simulink model "REL_TestModel"  (R2022a)
settings: Solver=FixedStepDiscrete  StartTime=0.0  StopTime=10.0  FixedStep=0.01  RelTol=1e-3
settings Model: DataDictionary=DHM.sldd  Creator=DELL  LastModifiedBy=DELL
settings DataIOCC: SaveFormat=StructureWithTime
settings OptimizationCC: DefaultParameterBehavior=Inlined  EnhancedBackFolding=on  PassReuseOutputArgsAs=Individual arguments  ZeroExternalMemoryAtStartup=off  ZeroInternalMemoryAtStartup=off  OptimizeBlockOrder=speed  DifferentSizesBufferReuse=on  OptimizationCustomize=off  EfficientTunableParamExpr=on
settings DebuggingCC: ParameterTunabilityLossMsg=error
settings ModelReferenceCC: ModelReferenceNumInstancesAllowed=Single
settings SFSimCC: MATLABDynamicMemAlloc=off
settings RTWCC: Description=AUTOSAR  SystemTargetFile=autosar.tlc  GenCodeOnly=on  TemplateMakefile=ert_default_tmf
settings CodeAppCC: ForceParamTrailComments=on  IgnoreCustomStorageClasses=off  OperatorAnnotations=on  SimulinkDataObjDesc=on  SFDataObjDesc=on  InsertBlockDesc=on
settings STFCustomTargetCC: TargetLangStandard=C99 (ISO)  MultiwordLength=256  ParMdlRefBuildCompliant=on  CompOptLevelCompliant=on  IncludeMdlTerminateFcn=off  CombineOutputUpdateFcns=on  SuppressErrorStatus=on  ERTCustomFileBanners=on  SupportNonFinite=off  SupportComplex=off  SupportContinuousTime=off  SupportNonInlinedSFcns=off  RemoveResetFunc=on  MATLABClassNameForMDSCustomization=Simulink.SoftwareTarget.ERTCustomization  AutosarCompliant=on  GRTInterface=off  UseToolchainInfoCompliant=on  LookupTableObjectStructAxisOrder=2,1,3,4,...  LUTObjectStructOrderEvenSpacing=Size,Table,Breakpoints  SystemTargetFile=autosar.tlc
settings ERTTargetCC: TargetLangStandard=C99 (ISO)  ConcurrentExecutionCompliant=off  IncludeMdlTerminateFcn=off  SuppressErrorStatus=on  SupportNonFinite=off  SupportComplex=off  ModelStepFunctionPrototypeControlCompliant=off  CPPClassGenCompliant=off  AutosarCompliant=on  LookupTableObjectStructAxisOrder=2,1,3,4,...  LUTObjectStructOrderEvenSpacing=Size,Table,Breakpoints  InlinedParameterPlacement=NonHierarchical  ERTCustomFileTemplate=example_file_process.tlc

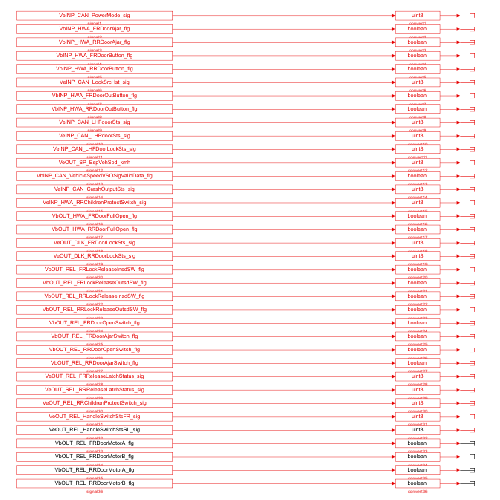
[thumbnail: Simulink's stored preview of the top-level diagram]
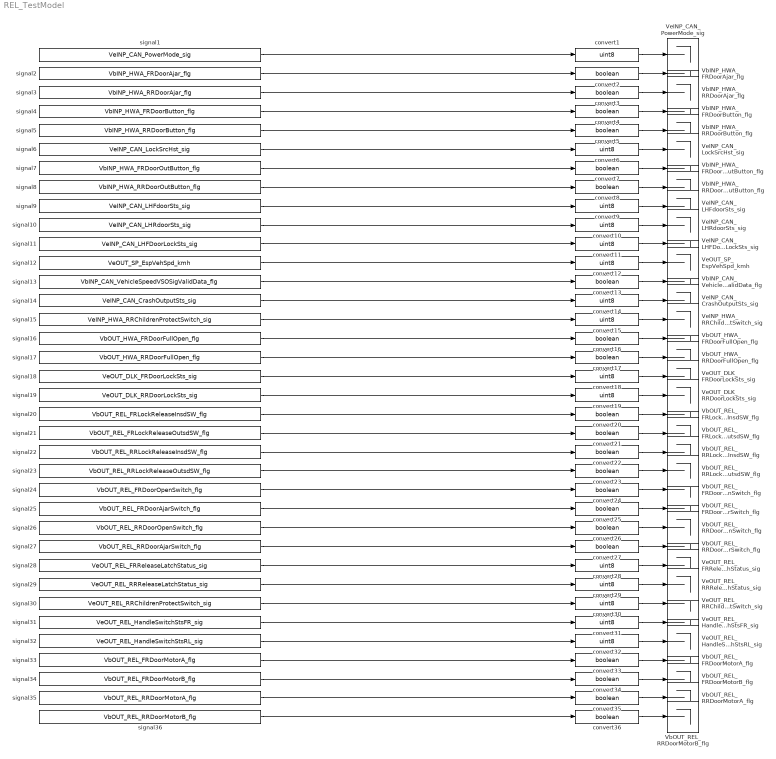
== system REL_TestModel ==
  VbINP_CAN_VehicleSpeedVSOSigValidData_flg : Terminator
  VbINP_HWA_FRDoorAjar_flg : Terminator
  VbINP_HWA_FRDoorButton_flg : Terminator
  VbINP_HWA_FRDoorOutButton_flg : Terminator
  VbINP_HWA_RRDoorAjar_flg : Terminator
  VbINP_HWA_RRDoorButton_flg : Terminator
  VbINP_HWA_RRDoorOutButton_flg : Terminator
  VbOUT_HWA_FRDoorFullOpen_flg : Terminator
  VbOUT_HWA_RRDoorFullOpen_flg : Terminator
  VbOUT_REL_FRDoorAjarSwitch_flg : Terminator
  VbOUT_REL_FRDoorMotorA_flg : Terminator
  VbOUT_REL_FRDoorMotorB_flg : Terminator
  VbOUT_REL_FRDoorOpenSwitch_flg : Terminator
  VbOUT_REL_FRLockReleaseInsdSW_flg : Terminator
  VbOUT_REL_FRLockReleaseOutsdSW_flg : Terminator
  VbOUT_REL_RRDoorAjarSwitch_flg : Terminator
  VbOUT_REL_RRDoorMotorA_flg : Terminator
  VbOUT_REL_RRDoorMotorB_flg : Terminator
  VbOUT_REL_RRDoorOpenSwitch_flg : Terminator
  VbOUT_REL_RRLockReleaseInsdSW_flg : Terminator
  VbOUT_REL_RRLockReleaseOutsdSW_flg : Terminator
  VeINP_CAN_CrashOutputSts_sig : Terminator
  VeINP_CAN_LHFDoorLockSts_sig : Terminator
  VeINP_CAN_LHFdoorSts_sig : Terminator
  VeINP_CAN_LHRdoorSts_sig : Terminator
  VeINP_CAN_LockSrcHst_sig : Terminator
  VeINP_CAN_PowerMode_sig : Terminator
  VeINP_HWA_RRChildrenProtectSwitch_sig : Terminator
  VeOUT_DLK_FRDoorLockSts_sig : Terminator
  VeOUT_DLK_RRDoorLockSts_sig : Terminator
  VeOUT_REL_FRReleaseLatchStatus_sig : Terminator
  VeOUT_REL_HandleSwitchStsFR_sig : Terminator
  VeOUT_REL_HandleSwitchStsRL_sig : Terminator
  VeOUT_REL_RRChildrenProtectSwitch_sig : Terminator
  VeOUT_REL_RRReleaseLatchStatus_sig : Terminator
  VeOUT_SP_EspVehSpd_kmh : Terminator
  convert{1,6,9..12,14..15,18..19,28..32} (15 alike) : DataTypeConversion  OutDataTypeStr=uint8  SaturateOnIntegerOverflow=off  RndMeth=Floor
  convert{2..5,7..8,13,16..17,20..27,33..36} (21 alike) : DataTypeConversion  OutDataTypeStr=boolean  SaturateOnIntegerOverflow=off  RndMeth=Floor
  signal1 : FromWorkspace  VariableName=VeINP_CAN_PowerMode_sig  SampleTime=-1  Interpolate=off  OutputAfterFinalValue=Holding final value
  signal10 : FromWorkspace  VariableName=VeINP_CAN_LHRdoorSts_sig  SampleTime=-1  Interpolate=off  OutputAfterFinalValue=Holding final value
  signal11 : FromWorkspace  VariableName=VeINP_CAN_LHFDoorLockSts_sig  SampleTime=-1  Interpolate=off  OutputAfterFinalValue=Holding final value
  signal12 : FromWorkspace  VariableName=VeOUT_SP_EspVehSpd_kmh  SampleTime=-1  Interpolate=off  OutputAfterFinalValue=Holding final value
  signal13 : FromWorkspace  VariableName=VbINP_CAN_VehicleSpeedVSOSigValidData_flg  SampleTime=-1  Interpolate=off  OutputAfterFinalValue=Holding final value
  signal14 : FromWorkspace  VariableName=VeINP_CAN_CrashOutputSts_sig  SampleTime=-1  Interpolate=off  OutputAfterFinalValue=Holding final value
  signal15 : FromWorkspace  VariableName=VeINP_HWA_RRChildrenProtectSwitch_sig  SampleTime=-1  Interpolate=off  OutputAfterFinalValue=Holding final value
  signal16 : FromWorkspace  VariableName=VbOUT_HWA_FRDoorFullOpen_flg  SampleTime=-1  Interpolate=off  OutputAfterFinalValue=Holding final value
  signal17 : FromWorkspace  VariableName=VbOUT_HWA_RRDoorFullOpen_flg  SampleTime=-1  Interpolate=off  OutputAfterFinalValue=Holding final value
  signal18 : FromWorkspace  VariableName=VeOUT_DLK_FRDoorLockSts_sig  SampleTime=-1  Interpolate=off  OutputAfterFinalValue=Holding final value
  signal19 : FromWorkspace  VariableName=VeOUT_DLK_RRDoorLockSts_sig  SampleTime=-1  Interpolate=off  OutputAfterFinalValue=Holding final value
  signal2 : FromWorkspace  VariableName=VbINP_HWA_FRDoorAjar_flg  SampleTime=-1  Interpolate=off  OutputAfterFinalValue=Holding final value
  signal20 : FromWorkspace  VariableName=VbOUT_REL_FRLockReleaseInsdSW_flg  SampleTime=-1  Interpolate=off  OutputAfterFinalValue=Holding final value
  signal21 : FromWorkspace  VariableName=VbOUT_REL_FRLockReleaseOutsdSW_flg  SampleTime=-1  Interpolate=off  OutputAfterFinalValue=Holding final value
  signal22 : FromWorkspace  VariableName=VbOUT_REL_RRLockReleaseInsdSW_flg  SampleTime=-1  Interpolate=off  OutputAfterFinalValue=Holding final value
  signal23 : FromWorkspace  VariableName=VbOUT_REL_RRLockReleaseOutsdSW_flg  SampleTime=-1  Interpolate=off  OutputAfterFinalValue=Holding final value
  signal24 : FromWorkspace  VariableName=VbOUT_REL_FRDoorOpenSwitch_flg  SampleTime=-1  Interpolate=off  OutputAfterFinalValue=Holding final value
  signal25 : FromWorkspace  VariableName=VbOUT_REL_FRDoorAjarSwitch_flg  SampleTime=-1  Interpolate=off  OutputAfterFinalValue=Holding final value
  signal26 : FromWorkspace  VariableName=VbOUT_REL_RRDoorOpenSwitch_flg  SampleTime=-1  Interpolate=off  OutputAfterFinalValue=Holding final value
  signal27 : FromWorkspace  VariableName=VbOUT_REL_RRDoorAjarSwitch_flg  SampleTime=-1  Interpolate=off  OutputAfterFinalValue=Holding final value
  signal28 : FromWorkspace  VariableName=VeOUT_REL_FRReleaseLatchStatus_sig  SampleTime=-1  Interpolate=off  OutputAfterFinalValue=Holding final value
  signal29 : FromWorkspace  VariableName=VeOUT_REL_RRReleaseLatchStatus_sig  SampleTime=-1  Interpolate=off  OutputAfterFinalValue=Holding final value
  signal3 : FromWorkspace  VariableName=VbINP_HWA_RRDoorAjar_flg  SampleTime=-1  Interpolate=off  OutputAfterFinalValue=Holding final value
  signal30 : FromWorkspace  VariableName=VeOUT_REL_RRChildrenProtectSwitch_sig  SampleTime=-1  Interpolate=off  OutputAfterFinalValue=Holding final value
  signal31 : FromWorkspace  VariableName=VeOUT_REL_HandleSwitchStsFR_sig  SampleTime=-1  Interpolate=off  OutputAfterFinalValue=Holding final value
  signal32 : FromWorkspace  VariableName=VeOUT_REL_HandleSwitchStsRL_sig  SampleTime=-1  Interpolate=off  OutputAfterFinalValue=Holding final value
  signal33 : FromWorkspace  VariableName=VbOUT_REL_FRDoorMotorA_flg  SampleTime=-1  Interpolate=off  OutputAfterFinalValue=Holding final value
  signal34 : FromWorkspace  VariableName=VbOUT_REL_FRDoorMotorB_flg  SampleTime=-1  Interpolate=off  OutputAfterFinalValue=Holding final value
  signal35 : FromWorkspace  VariableName=VbOUT_REL_RRDoorMotorA_flg  SampleTime=-1  Interpolate=off  OutputAfterFinalValue=Holding final value
  signal36 : FromWorkspace  VariableName=VbOUT_REL_RRDoorMotorB_flg  SampleTime=-1  Interpolate=off  OutputAfterFinalValue=Holding final value
  signal4 : FromWorkspace  VariableName=VbINP_HWA_FRDoorButton_flg  SampleTime=-1  Interpolate=off  OutputAfterFinalValue=Holding final value
  signal5 : FromWorkspace  VariableName=VbINP_HWA_RRDoorButton_flg  SampleTime=-1  Interpolate=off  OutputAfterFinalValue=Holding final value
  signal6 : FromWorkspace  VariableName=VeINP_CAN_LockSrcHst_sig  SampleTime=-1  Interpolate=off  OutputAfterFinalValue=Holding final value
  signal7 : FromWorkspace  VariableName=VbINP_HWA_FRDoorOutButton_flg  SampleTime=-1  Interpolate=off  OutputAfterFinalValue=Holding final value
  signal8 : FromWorkspace  VariableName=VbINP_HWA_RRDoorOutButton_flg  SampleTime=-1  Interpolate=off  OutputAfterFinalValue=Holding final value
  signal9 : FromWorkspace  VariableName=VeINP_CAN_LHFdoorSts_sig  SampleTime=-1  Interpolate=off  OutputAfterFinalValue=Holding final value
  wires:
  signal1/1 -> convert1/1
  signal2/1 -> convert2/1
  signal3/1 -> convert3/1
  signal4/1 -> convert4/1
  signal5/1 -> convert5/1
  signal6/1 -> convert6/1
  signal7/1 -> convert7/1
  signal8/1 -> convert8/1
  signal9/1 -> convert9/1
  signal10/1 -> convert10/1
  signal11/1 -> convert11/1
  signal12/1 -> convert12/1
  signal13/1 -> convert13/1
  signal14/1 -> convert14/1
  signal15/1 -> convert15/1
  signal16/1 -> convert16/1
  signal17/1 -> convert17/1
  signal18/1 -> convert18/1
  signal19/1 -> convert19/1
  signal20/1 -> convert20/1
  signal21/1 -> convert21/1
  signal22/1 -> convert22/1
  signal23/1 -> convert23/1
  signal24/1 -> convert24/1
  signal25/1 -> convert25/1
  signal26/1 -> convert26/1
  signal27/1 -> convert27/1
  signal28/1 -> convert28/1
  signal29/1 -> convert29/1
  signal30/1 -> convert30/1
  signal31/1 -> convert31/1
  signal32/1 -> convert32/1
  signal33/1 -> convert33/1
  signal34/1 -> convert34/1
  signal35/1 -> convert35/1
  signal36/1 -> convert36/1
  convert1/1 -> VeINP_CAN_PowerMode_sig/1
  convert10/1 -> VeINP_CAN_LHRdoorSts_sig/1
  convert11/1 -> VeINP_CAN_LHFDoorLockSts_sig/1
  convert12/1 -> VeOUT_SP_EspVehSpd_kmh/1
  convert13/1 -> VbINP_CAN_VehicleSpeedVSOSigValidData_flg/1
  convert14/1 -> VeINP_CAN_CrashOutputSts_sig/1
  convert15/1 -> VeINP_HWA_RRChildrenProtectSwitch_sig/1
  convert16/1 -> VbOUT_HWA_FRDoorFullOpen_flg/1
  convert17/1 -> VbOUT_HWA_RRDoorFullOpen_flg/1
  convert18/1 -> VeOUT_DLK_FRDoorLockSts_sig/1
  convert19/1 -> VeOUT_DLK_RRDoorLockSts_sig/1
  convert2/1 -> VbINP_HWA_FRDoorAjar_flg/1
  convert20/1 -> VbOUT_REL_FRLockReleaseInsdSW_flg/1
  convert21/1 -> VbOUT_REL_FRLockReleaseOutsdSW_flg/1
  convert22/1 -> VbOUT_REL_RRLockReleaseInsdSW_flg/1
  convert23/1 -> VbOUT_REL_RRLockReleaseOutsdSW_flg/1
  convert24/1 -> VbOUT_REL_FRDoorOpenSwitch_flg/1
  convert25/1 -> VbOUT_REL_FRDoorAjarSwitch_flg/1
  convert26/1 -> VbOUT_REL_RRDoorOpenSwitch_flg/1
  convert27/1 -> VbOUT_REL_RRDoorAjarSwitch_flg/1
  convert28/1 -> VeOUT_REL_FRReleaseLatchStatus_sig/1
  convert29/1 -> VeOUT_REL_RRReleaseLatchStatus_sig/1
  convert3/1 -> VbINP_HWA_RRDoorAjar_flg/1
  convert30/1 -> VeOUT_REL_RRChildrenProtectSwitch_sig/1
  convert31/1 -> VeOUT_REL_HandleSwitchStsFR_sig/1
  convert32/1 -> VeOUT_REL_HandleSwitchStsRL_sig/1
  convert33/1 -> VbOUT_REL_FRDoorMotorA_flg/1
  convert34/1 -> VbOUT_REL_FRDoorMotorB_flg/1
  convert35/1 -> VbOUT_REL_RRDoorMotorA_flg/1
  convert36/1 -> VbOUT_REL_RRDoorMotorB_flg/1
  convert4/1 -> VbINP_HWA_FRDoorButton_flg/1
  convert5/1 -> VbINP_HWA_RRDoorButton_flg/1
  convert6/1 -> VeINP_CAN_LockSrcHst_sig/1
  convert7/1 -> VbINP_HWA_FRDoorOutButton_flg/1
  convert8/1 -> VbINP_HWA_RRDoorOutButton_flg/1
  convert9/1 -> VeINP_CAN_LHFdoorSts_sig/1
